simulink model "ObserverPhysical"  (R2021b)
settings: Solver=FixedStepAuto  StartTime=0.0  StopTime=RunTime  FixedStep=time_step  RelTol=1e-3  EnableMultiTasking=on
values from neighbouring files (symbols this model uses):
  adingain = [adin_gain 1 1 1 1 1]    [hwinit.m]
  adinoffs = [adin_offs 0 0 0 0 0]    [hwinit.m]
  daoutgain = 1*[-6]    [hwinit.m]
  daoutoffs = [0.00]    [hwinit.m]
  h = 0.001    [hwinit.m]
  Ke = [-470.433246005  -124.870251625; 109361.94636  30162.7836696; 1152.72458568  337.286863362; -229625.613509  -62717.5596066; -659483.424198  -193368.313296]    [ObserverMatrix.mat]
  theta_1_Op = pi    (= 3.14159265359)    [ObserverPhysical_script.m]
  theta_2_Op = x_operating(3)    [ObserverPhysical_script.m]
undefined symbols (not defined in the file or in its folder): A, B, C
settings Model: Creator=rbabuska  LastModifiedBy=amavanmierlo
settings SolverCC: AlgebraicLoopSolver=TrustRegion
settings DataIOCC: LimitDataPoints=on  SaveFormat=Array  ReturnWorkspaceOutputs=off  SignalLoggingName=sigsOut
settings OptimizationCC: BooleanDataType=off  ExpressionDepthLimit=2147483647  InitFltsAndDblsToZero=on  LifeSpan=inf
settings DebuggingCC: SaveWithParameterizedLinksMsg=none  SignalResolutionControl=TryResolveAllWithWarning  MultiTaskDSMMsg=warning  MultiTaskCondExecSysMsg=none  AllowSymbolicDim=off  StateNameClashWarn=warning  SFUnexpectedBacktrackingDiag=warning  SFNoUnconditionalDefaultTransitionDiag=warning  SFExecutionAtInitializationDiag=none  SFMachineParentedDataDiag=warning  ArithmeticOperatorsInVariantConditions=warning
settings HardwareCC: ProdBitPerPointer=32  ProdBitPerSizeT=32  ProdBitPerPtrDiffT=32  ProdLargestAtomicFloat=None  ProdIntDivRoundTo=Undefined  ProdEndianess=Unspecified  ProdWordSize=32  ProdHWDeviceType=32-bit Generic  TargetUnknown=on
settings ModelReferenceCC: PropagateSignalLabelsOutOfModel=off
settings SFSimCC: SimUseLocalCustomCode=off  CustomCodeUndefinedFunction=UseInterfaceOnly
settings RTWCC: RTWUseLocalCustomCode=off
settings CodeAppCC: StateflowObjectComments=on
settings GRTTargetCC: TargetFcnLib=ansi_tfl_tmw.mat  TargetLangStandard=C89/C90 (ANSI)  CombineOutputUpdateFcns=off  GRTInterface=on
settings ConfigComp: CovMetricSettings=dw  CovSaveCumulativeToWorkspaceVar=on  CovSaveSingleToWorkspaceVar=on  CovExternalEMLEnable=off

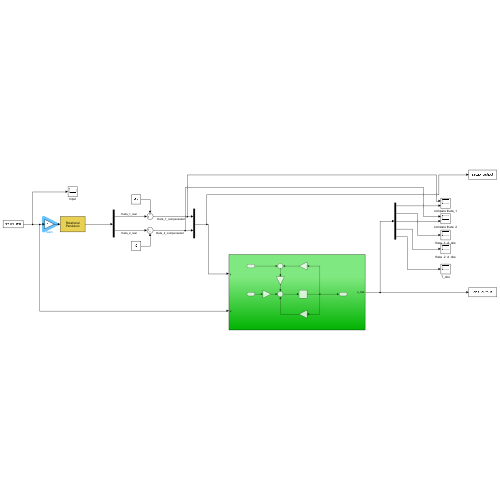
[thumbnail: Simulink's stored preview of the top-level diagram]
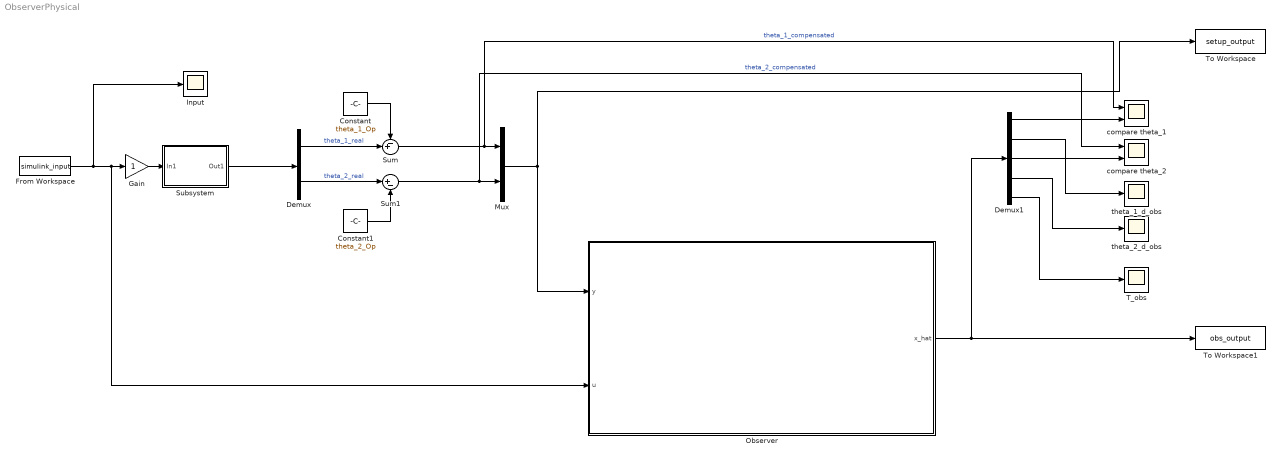
== system ObserverPhysical ==
  Constant : Constant  Value=theta_1_Op
  Constant1 : Constant  Value=theta_2_Op
  Demux : Demux  Outputs=2
  Demux1 : Demux  Outputs=5
  From Workspace : FromWorkspace  SampleTime=-1
  Gain : Gain
  Input : Scope
  Mux : Mux  Inputs=2
  Observer : Subsystem
  Subsystem : Subsystem
      mask Display: disp('Rotational\nPendulum')
  Sum : Sum  Inputs=-+|
  Sum1 : Sum  Inputs=|+-
  T_obs : Scope
  To Workspace : ToWorkspace  VariableName=setup_output  SaveFormat=Timeseries  SampleTime=-1
  To Workspace1 : ToWorkspace  VariableName=obs_output  SaveFormat=Timeseries  SampleTime=-1
  compare theta_1 : Scope  NumInputPorts=2
  compare theta_2 : Scope  NumInputPorts=2
  theta_1_d_obs : Scope
  theta_2_d_obs : Scope
  wires:
  From Workspace/1 -> Observer/2(u), Gain/1, Input/1
  Demux/1 -> Sum/2  "theta_1_real"
  Demux/2 -> Sum1/1  "theta_2_real"
  Subsystem/1(Out1) -> Demux/1
  Mux/1 -> To Workspace/1, Observer/1(y)
  Sum1/1 -> compare theta_2/1, Mux/2  "theta_2_compensated"
  Sum/1 -> Mux/1, compare theta_1/1  "theta_1_compensated"
  Constant/1 -> Sum/1
  Constant1/1 -> Sum1/2
  Observer/1(x_hat) -> To Workspace1/1, Demux1/1
  Demux1/3 -> compare theta_2/2
  Demux1/1 -> compare theta_1/2
  Demux1/2 -> theta_1_d_obs/1
  Demux1/5 -> T_obs/1
  Demux1/4 -> theta_2_d_obs/1
  Gain/1 -> Subsystem/1(In1)

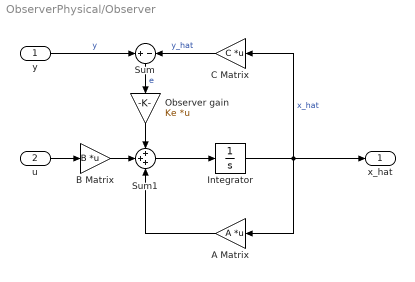
== system ObserverPhysical/Observer ==
  y : Inport
  u : Inport  Port=2
  A Matrix : Gain  Gain=A  Multiplication=Matrix(K*u)
  B Matrix : Gain  Gain=B  Multiplication=Matrix(K*u)
  C Matrix : Gain  Gain=C  Multiplication=Matrix(K*u)
  Integrator : Integrator
  Observer gain : Gain  Gain=Ke  Multiplication=Matrix(K*u)
  Sum : Sum  Inputs=+|-
  Sum1 : Sum  Inputs=+++
  x_hat : Outport
  wires:
  Integrator/1 -> C Matrix/1, A Matrix/1, x_hat/1  "x_hat"
  y/1 -> Sum/1  "y"
  C Matrix/1 -> Sum/2  "y_hat"
  Sum1/1 -> Integrator/1
  Sum/1 -> Observer gain/1  "e"
  Observer gain/1 -> Sum1/1
  A Matrix/1 -> Sum1/3
  B Matrix/1 -> Sum1/2
  u/1 -> B Matrix/1

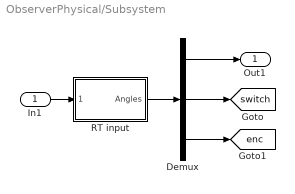
== system ObserverPhysical/Subsystem ==
  In1 : Inport
  Demux : Demux  Outputs=[2 4 1]
  RT input : Subsystem  mask{Ts=h, channels=[6 7]}
      mask prompts: Ts "Sample time [s]:"; channels "Channels to read (e.g., [6 7])"
      mask init:
      | hwinit;
      | 
      | % initialize FPGA
      | fugihandle = fugiboard('Open', 'Pendulum1');
      | fugihandle.WatchdogTimeout = 0.5;
      | fugiboard('SetParams', fugihandle);
      | fugiboard('Write', fugihandle, 0, 0, 0, 0);  % dummy write to sync interface board
      | fugiboard('Write', fugihandle, 5, 1, 0, 0);  % reset position, activate relay
      | data = fugiboard('Read', fugihandle);        % get version info from FPGA
      | % model = bitshift(data(1), -5); 
      | % version = bitand(data(1), 31);
      | % disp(sprintf('FPGA setup %d, version %d', model, version)); % for the B&P it should say 1 1, or else there is a problem
      | fugiboard('Write', fugihandle, 0, 1, 0, 0);  % end reset
      | pause(0.1);                         % give relay some time to respond
      mask Display: disp('Rotational\nPendulum')
  Out1 : Outport
  tag scope: enc=global, switch=global
  wires:
  RT input/1(Angles) -> Demux/1
  Demux/1 -> Out1/1
  Demux/2 -> [switch]
  Demux/3 -> [enc]
  In1/1 -> RT input/1(Motors)

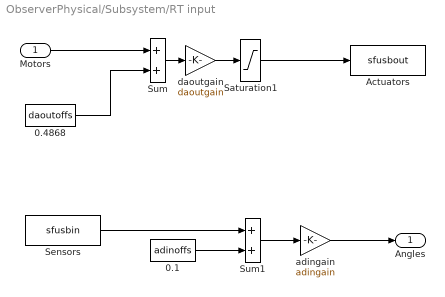
== system ObserverPhysical/Subsystem/RT input ==
  Motors : Inport
  0.1 : Constant  Value=adinoffs
  0.4868 : Constant  Value=daoutoffs
  Actuators : S-Function  FunctionName=sfusbout  Parameters=Ts, fugihandle  SFunctionDeploymentMode=off  EnableBusSupport=off
  Saturation1 : Saturate  UpperLimit=10  LowerLimit=-10
  Sensors : S-Function  FunctionName=sfusbin  Parameters=Ts, fugihandle, channels  SFunctionDeploymentMode=off  EnableBusSupport=off
  Sum : Sum  InputSameDT=on  SaturateOnIntegerOverflow=on  OutDataTypeStr=Inherit: Same as first input
  Sum1 : Sum  InputSameDT=on  SaturateOnIntegerOverflow=on  OutDataTypeStr=Inherit: Same as first input
  adingain : Gain  Gain=adingain  SaturateOnIntegerOverflow=on  OutDataTypeStr=Inherit: Same as input  ParamDataTypeStr=Inherit: Same as input
  daoutgain : Gain  Gain=daoutgain  SaturateOnIntegerOverflow=on  OutDataTypeStr=Inherit: Same as input  ParamDataTypeStr=Inherit: Same as input
  Angles : Outport
  wires:
  Sum/1 -> daoutgain/1
  0.4868/1 -> Sum/2
  Motors/1 -> Sum/1
  Sum1/1 -> adingain/1
  0.1/1 -> Sum1/2
  adingain/1 -> Angles/1
  Saturation1/1 -> Actuators/1
  daoutgain/1 -> Saturation1/1
  Sensors/1 -> Sum1/1
